simulink model "Microgrid202510141004"  (R2025a)
settings: Solver=ode23tb  StartTime=0  StopTime=2592000  FixedStep=3600  MaxStep=3600  MinStep=1e-4  RelTol=1e-4  AbsTol=1e-6
StartFcn:
  | fprintf('=== Starting Episode [%s] ===\n', datestr(now, 'HH:MM:SS'));
undefined symbols (not defined in the file): D1, Delta
libraries: spsThreePhaseDynamicLoadLib x3, fuzblock x2, spsThreePhaseVIMeasurementLib x2, simulink x1, spsThreePhaseSeriesRLCLoadLib x1, rllib x1, spsThreePhaseTransformerTwoWindingsLib x1, spsThreePhaseBreakerLib x1, spsThreePhaseSourceLib x1, sps_lib x1
settings Model: DataTypeOverride=Off  Creator=jlesage  LastModifiedBy=86138
settings SolverCC: InitialStep=0.1  ZcThreshold=1e-12  AlgebraicLoopSolver=TrustRegion
settings DataIOCC: SaveState=on  ReturnWorkspaceOutputs=off
settings OptimizationCC: OptimizeBlockIOStorage=off  OptimizeDataStoreBuffers=off  BusAssignmentInplaceUpdate=off
settings DebuggingCC: SigSpecEnsureSampleTimeMsg=none  SFUnexpectedBacktrackingDiag=warning  SFNoUnconditionalDefaultTransitionDiag=warning  ArithmeticOperatorsInVariantConditions=warning
settings ModelReferenceCC: EnableRefExpFcnMdlSchedulingChecks=on
settings SFSimCC: SimUseLocalCustomCode=off  CustomCodeUndefinedFunction=UseInterfaceOnly
settings RTWCC: GenCodeOnly=on  GenerateReport=on  RTWUseLocalCustomCode=off  BuildConfiguration=Debug  LaunchReport=on  GPUComputeCapability=3.5
settings CodeAppCC: ForceParamTrailComments=on  MATLABSourceComments=on  EnableCustomComments=on
settings GRTTargetCC: MultiInstanceErrorCode=Warning  CombineSignalStateStructs=on  SupportVariableSizeSignals=on

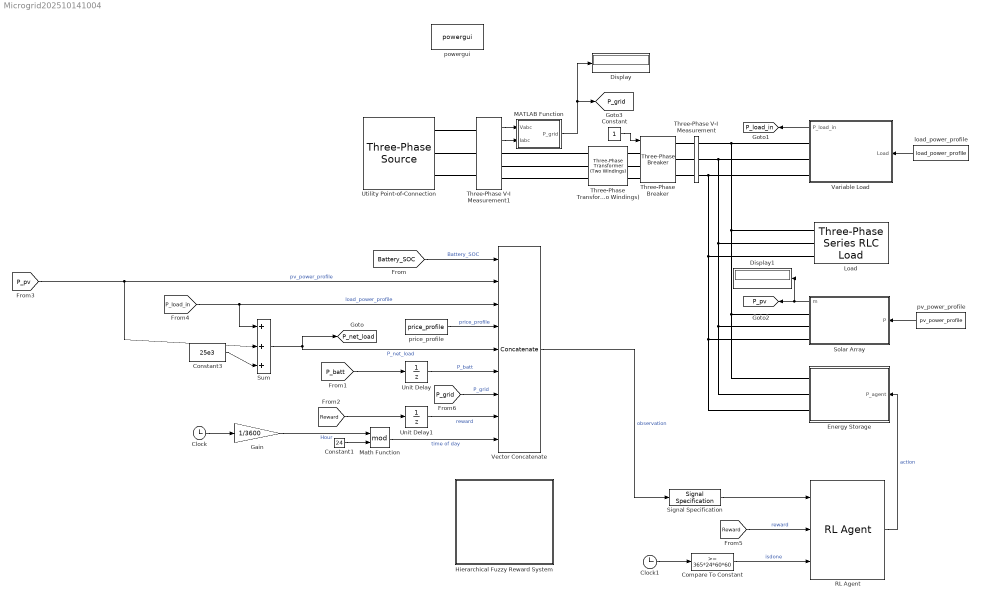
== system Microgrid202510141004 ==
  Clock : Clock
  Clock1 : Clock
  Compare To Constant : simulink/Logic and Bit Operations/Compare To Constant  relop=>=  const=365*24*60*60  OutDataTypeStr=boolean
  Constant : Constant
  Constant1 : Constant  Value=24
  Constant3 : Constant  Value=25e3
  Display : Display
  Display1 : Display
  Energy Storage : Subsystem  mask{Capacity_Ah=280, Fn=60, Vn=400}
      mask prompts: Capacity_Ah "Capacity_Ah of Battery"; Fn "Nominal Frequency [Hz]"; Vn "Nominal L-L Voltage [Vrms]"
      mask DialogControl ParameterGroupVar Prompt: 参数
  Gain : Gain  Gain=1/3600
  Hierarchical Fuzzy Reward System : Subsystem
  Load : spsThreePhaseSeriesRLCLoadLib/Three-Phase Series RLC Load  LConnTagsString=A|B|C  Configuration=Y (grounded)  NominalVoltage=400  Vabc=[1e3 1e3 1e3]  Vabcp=[1e3 1e3 1e3]  NominalFrequency=60  UnbalancedPower=off  ActivePower=25e3  InductivePower=0  CapacitivePower=0  Pabc=[10e3 9e3 11e3]  QLabc=[100 90 110]  QCabc=[100 90 110]  Pabcp=[10e3 9e3 11e3]  QLabcp=[100 90 110]  QCabcp=[100 90 110]  Measurements=None  LoadType=constant Z
      settings: AttributesFormatString=P = %<ActivePower> W
  MATLAB Function : MATLAB Function  TreatAsAtomicUnit=on
  Math Function : Math  Operator=mod
  RL Agent : rllib/RL Agent  Agent=agentObj  ExternalActionAsInput=off  ProvideLastAction=off  ProvideCumRwd=off  TreatAsDirectFeedthrough=on  UseStrictObservationDataTypes=off
  Signal Specification : SignalSpecification  Dimensions=9  SampleTime=3600
  Solar Array : Subsystem  mask(Grid-Connected PV Array (PQ Model)){Vn=400, Fn=60}
      mask prompts: Vn "Nominal L-L Voltage [Vrms]"; Fn "Nominal Frequency [Hz]"
      mask help:
      | This block models a grid-connected solar array using the Three-Phase Dynamic Load block. This is a system-level model that does not contain any power electronics, but is useful for load flow, phasor, and hybrid phasor-EMT simulations. The input to this block is the power output of the grid connected PV array, not irradiance.
      |
      | For more detailed PV models, consider the PV Array block in the Renewables library. Consider using this PQ Model to perform load flow studies and switch to a more detailed model when full EMT studies are required.
      |
      | Note: The array power must be specified for use for Load Flow analysis.
      mask Display:
      | color('white')
      | port_label('input',1,'P')
      | port_label('output',1,'m')
      | port_label('Rconn',1,'A')
      | port_label('Rconn',2,'B')
      | port_label('Rconn',3,'C')
  Sum : Sum  Inputs=+++|
  Three-Phase Transformer (Two Windings) : spsThreePhaseTransformerTwoWindingsLib/Three-Phase Transformer (Two Windings)  Winding1Connection=Delta (D1)  Winding2Connection=Yg  CoreType=Three single-phase transformers  SetSaturation=off  Hysteresis=off  DataFile='hysteresis'  SetInitialFlux=off  Measurements=None  UNITS=pu  NominalPower=[ 100e3, 60 ]  Winding1=[ 13.8e3 , 0.002 , 0.08 ]  Winding2=[ 400 , 0.002 , 0.08 ]  Rm=500  Lm=500  L0=0.5  Saturation=[ 0,0 ; 0.0024,1.2 ; 1.0,1.52 ]  InitialFluxes=[ 0.8 , -0.8 , 0.7 ]  BreakLoop=off  DiscreteSolver=Trapezoidal iterative  DataType=off  TransfoNumber=1
  Three-Phase V-I Measurement : spsThreePhaseVIMeasurementLib/Three-Phase V-I Measurement  VoltageMeasurement=phase-to-ground  SetLabelV=on  LabelV=Vabc  Vpu=off  VpuLL=off  CurrentMeasurement=yes  SetLabelI=on  LabelI=Iabc  Ipu=off  Pbase=100e6  Vbase=500e3  OutputType=Complex  PhasorSimulation=on  PSBequivalent=0
  Three-Phase V-I Measurement1 : spsThreePhaseVIMeasurementLib/Three-Phase V-I Measurement  VoltageMeasurement=phase-to-ground  SetLabelV=off  LabelV=Vabc  Vpu=off  VpuLL=off  CurrentMeasurement=yes  SetLabelI=off  LabelI=Iabc  Ipu=off  Pbase=100e6  Vbase=500e3  OutputType=Complex  PhasorSimulation=on  PSBequivalent=0
  Three-Phase Breaker : spsThreePhaseBreakerLib/Three-Phase Breaker  InitialState=closed  SwitchA=on  SwitchB=on  SwitchC=on  SwitchTimes="[1/60  5/60]"  External=on  BreakerResistance=0.01  SnubberResistance=1e6  SnubberCapacitance=inf  Measurements=None
  Unit Delay : UnitDelay  SampleTime=-1  HasFrameUpgradeWarning=on
  Unit Delay1 : UnitDelay  SampleTime=-1  HasFrameUpgradeWarning=on
  Utility Point-of-Connection : spsThreePhaseSourceLib/Three-Phase Source  InternalConnection=Yg  VoltagePhases=off  Voltage=(13800)*1.00243  PhaseAngle=0.071468  Voltage_phases=[25e3 25e3 25e3]/sqrt(3)  PhaseAngles_phases=[0 -120 +120]  Frequency=60  NonIdealSource=on  SpecifyImpedance=on  Resistance=0.8929  Inductance=16.58e-3  ShortCircuitLevel=250e6  BaseVoltage=13.8e3  XRratio=7  BusType=swing  Pref=10e3  Qref=0  Prefabc=[10e3, 10e3, 10e3]  Qrefabc=[0, 0, 0]  Qmin=-inf  Qmax=inf
  Variable Load : Subsystem  mask(Variable Load (PQ Model)){Vn=400, Fn=60}
      mask prompts: Vn "Nominal L-L Voltage [Vrms]"; Fn "Nominal Frequency [Hz]"
      mask help:
      | The Variable Load block is a lumped approximation for a distribution feeder. For non-unity power factor loads, the input (active power) is scaled accordingly to generate a desired load.
      |
      | Note: The initial input load must be specified for use for Load Flow analysis.
      mask Display:
      | color('white')
      | port_label('input',1,'Load')
      | port_label('Rconn',1,'A')
      | port_label('Rconn',2,'B')
      | port_label('Rconn',3,'C')
  Vector Concatenate : Concatenate  NumInputs=9
  load_power_profile : FromWorkspace  VariableName=load_power_profile  SampleTime=3600
  powergui : sps_lib/powergui  Priority=1  SimulationMode=Phasor  SampleTime=1e-4  frequency=60  Iterations=50  frequencyindice=60  Pbase=100e6  ErrMax=0.0001  UnitsV=kV  UnitsW=MW  buscounter=3  FunctionMessages=off  echomessages=off  EnableUseOfTLC=off  CurrentSourceSwitches=off  DisableSnubberDevices=off  DisableRonSwitches=off  DisableVfSwitches=off  DisplayEquations=off  AutomaticDiscreteSolvers=off  SolverType=Tustin/Backward Euler (TBE)  Interpol=off  ExternalGateDelay=off  methode=off  Ts=100  x0status=blocks  SPID=on  SwTol=0  HookPort=off  NonlinearTolerance=1e-4  nMaxIteration=100  ContinueOnMaxIteration=off  RestoreLinks=warning  ResistiveCurrentMeasurement=off  Frange=[0:2:500]  Ylog=off  Xlog=on  ShowGrid=off  save=off  variable=ZData  structure=0  ZoomFFT=off  StartTime=0.0  cycles=1  DisplayStyle=1  fundamental=60  FreqAxis=off  MaxFrequency=1000  frequencyindicesteady=1  RmsSteady=1  display=off
  price_profile : FromWorkspace  VariableName=price_profile  SampleTime=3600
  pv_power_profile : FromWorkspace  VariableName=pv_power_profile  SampleTime=3600
  tag scope: P_grid=global, P_load_in=global, P_net_load=global, P_pv=global
  wires:
  Constant/1 -> Three-Phase Breaker/1
  pv_power_profile/1 -> Solar Array/1(P)
  load_power_profile/1 -> Variable Load/1(Load)
  Solar Array/1(m) -> [P_pv], Display1/1
  Vector Concatenate/1 -> Signal Specification/1  "observation"
  Clock/1 -> Gain/1
  [Reward] -> RL Agent/2  "reward"
  Compare To Constant/1 -> RL Agent/3  "isdone"
  Clock1/1 -> Compare To Constant/1
  price_profile/1 -> Vector Concatenate/4  "price_profile"
  Gain/1 -> Math Function/1  "Hour"
  [Battery_SOC] -> Vector Concatenate/1  "Battery_SOC"
  [P_pv] -> Sum/2, Vector Concatenate/2  "pv_power_profile"
  [P_load_in] -> Sum/1, Vector Concatenate/3  "load_power_profile"
  Sum/1 -> Vector Concatenate/5, [P_net_load]  "P_net_load"
  [P_batt] -> Unit Delay/1
  [Reward] -> Unit Delay1/1
  Math Function/1 -> Vector Concatenate/9  "time of day"
  Constant1/1 -> Math Function/2
  Unit Delay1/1 -> Vector Concatenate/8  "reward"
  Constant3/1 -> Sum/3
  Variable Load/1(P_load_in) -> [P_load_in]
  Three-Phase V-I Measurement1/1 -> MATLAB Function/1(Vabc)
  Three-Phase V-I Measurement1/2 -> MATLAB Function/2(Iabc)
  MATLAB Function/1(P_grid) -> Display/1, [P_grid]
  Unit Delay/1 -> Vector Concatenate/6  "P_batt"
  [P_grid] -> Vector Concatenate/7  "P_grid"
  Signal Specification/1 -> RL Agent/1
  RL Agent/1 -> Energy Storage/1(P_agent)  "action"
  connections:
  Three-Phase Transformer (Two Windings)/RConn1 -- Three-Phase Breaker/LConn1
  Three-Phase Transformer (Two Windings)/RConn2 -- Three-Phase Breaker/LConn2
  Three-Phase Transformer (Two Windings)/RConn3 -- Three-Phase Breaker/LConn3
  Load/LConn1 -- Three-Phase V-I Measurement/RConn1 -- Variable Load/RConn1 -- Energy Storage/RConn1 -- Solar Array/RConn1
  Load/LConn2 -- Three-Phase V-I Measurement/RConn2 -- Variable Load/RConn2 -- Energy Storage/RConn2 -- Solar Array/RConn2
  Load/LConn3 -- Three-Phase V-I Measurement/RConn3 -- Variable Load/RConn3 -- Energy Storage/RConn3 -- Solar Array/RConn3
  Three-Phase Breaker/RConn1 -- Three-Phase V-I Measurement/LConn1
  Three-Phase Breaker/RConn2 -- Three-Phase V-I Measurement/LConn2
  Three-Phase Breaker/RConn3 -- Three-Phase V-I Measurement/LConn3
  Three-Phase V-I Measurement1/LConn1 -- Utility Point-of-Connection/RConn1
  Three-Phase V-I Measurement1/LConn2 -- Utility Point-of-Connection/RConn2
  Three-Phase V-I Measurement1/LConn3 -- Utility Point-of-Connection/RConn3
  Three-Phase V-I Measurement1/RConn3 -- Three-Phase Transformer (Two Windings)/LConn3
  Three-Phase V-I Measurement1/RConn2 -- Three-Phase Transformer (Two Windings)/LConn2
  Three-Phase V-I Measurement1/RConn1 -- Three-Phase Transformer (Two Windings)/LConn1

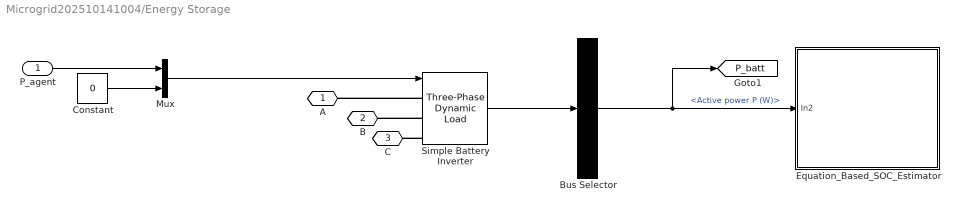
== system Microgrid202510141004/Energy Storage ==
  P_agent : Inport
  Bus Selector : BusSelector  OutputSignals=Active power P (W)
  Constant : Constant  Value=0
  Equation_Based_SOC_Estimator : Subsystem
  Mux : Mux  Inputs=2
  Simple Battery Inverter : spsThreePhaseDynamicLoadLib/Three-Phase Dynamic Load  NominalVoltage=[Vn Fn]  ActiveReactivePowers=[-100000 -3.38813e-13]  PositiveSequence=[0.999844 -0.0038635]  ExternalControl=on  NpNq=[1.3 2]  TimeConstants="[0  0  0  0]"  MinimumVoltage=0.7  Tfilter=1e-2  LoadFlowParameters=[4,0,0,0,0]
      settings: LibrarySourceBlock=|
      | sps_lib/Passives/Three-Phase
      | Dynamic Load
  A : PMIOPort  Side=Right
  B : PMIOPort  Port=2  Side=Right
  C : PMIOPort  Port=3  Side=Right
  tag scope: P_batt=global
  wires:
  Simple Battery Inverter/1 -> Bus Selector/1
  Bus Selector/1 -> [P_batt], Equation_Based_SOC_Estimator/1(In2)  "<Active power P (W)>"
  Mux/1 -> Simple Battery Inverter/1
  P_agent/1 -> Mux/1
  Constant/1 -> Mux/2
  connections:
  Simple Battery Inverter/LConn1 -- A/RConn1
  Simple Battery Inverter/LConn2 -- B/RConn1
  Simple Battery Inverter/LConn3 -- C/RConn1

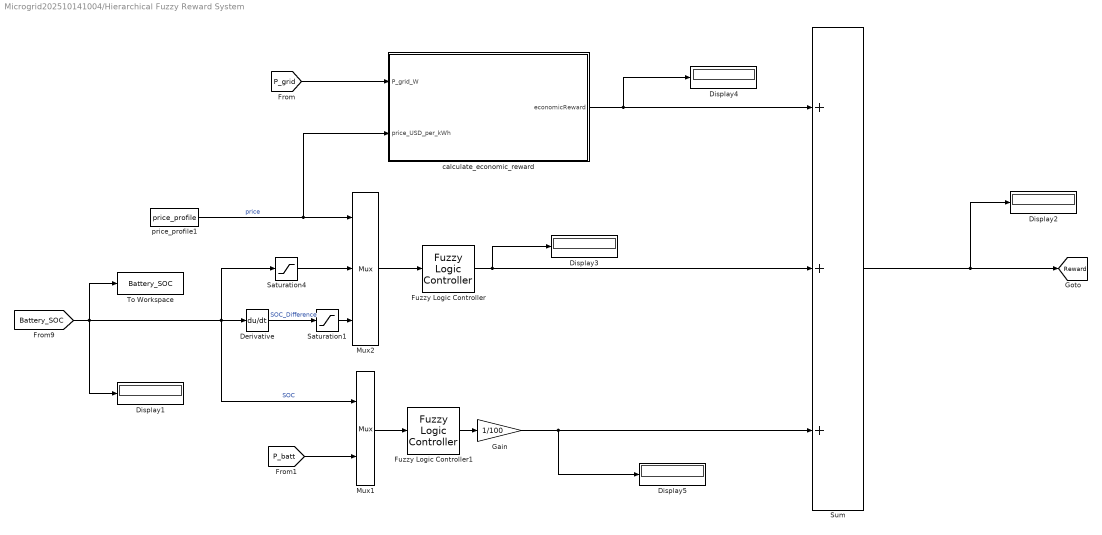
== system Microgrid202510141004/Hierarchical Fuzzy Reward System ==
  Derivative : Derivative
  Display{1..5} (5 alike) : Display
  Fuzzy Logic Controller : fuzblock/Fuzzy Logic  Controller  FIS='Battery_State_Type2.fis'  OutputSampleNumber=101  DataType=double  UseLookupTable=off  NumBreakpoints=10  FuzzifiedInputs=off  RuleFiringStrengths=off  RuleOutputs=off  AggregatedOutputs=off  SimulateUsing=Interpreted execution  OutOfRangeInputValueMessage=warning  NoRuleFiredMessage=warning  EmptyOutputFuzzySetMessage=warning
  Fuzzy Logic Controller1 : fuzblock/Fuzzy Logic  Controller  FIS='SOCProtector_Type2.fis'  OutputSampleNumber=101  DataType=double  UseLookupTable=off  NumBreakpoints=10  FuzzifiedInputs=off  RuleFiringStrengths=off  RuleOutputs=off  AggregatedOutputs=off  SimulateUsing=Interpreted execution  OutOfRangeInputValueMessage=warning  NoRuleFiredMessage=warning  EmptyOutputFuzzySetMessage=warning
  Gain : Gain  Gain=1/100
  Mux1 : Mux  Inputs=2
  Mux2 : Mux  Inputs=3
  Saturation1 : Saturate  UpperLimit=100  LowerLimit=-100  LinearizeAsGain=off  ZeroCross=off  OutMin=-100  RndMeth=Simplest
  Saturation4 : Saturate  UpperLimit=100  LowerLimit=0  LinearizeAsGain=off  ZeroCross=off  OutMin=0  RndMeth=Simplest
  Sum : Sum  Inputs=+++
  To Workspace : ToWorkspace  VariableName=Battery_SOC  SampleTime=3600
      settings: Save2DSignal=2-D array (concatenate along first dimension)
  calculate_economic_reward : MATLAB Function  TreatAsAtomicUnit=on
  price_profile1 : FromWorkspace  VariableName=price_profile
  tag scope: Reward=global
  wires:
  Sum/1 -> Display2/1, [Reward]
  Mux2/1 -> Fuzzy Logic Controller/1
  [Battery_SOC] -> Display1/1, To Workspace/1, Derivative/1, Mux1/1, Saturation4/1  "SOC"
  Derivative/1 -> Saturation1/1  "SOC_Difference"
  Saturation4/1 -> Mux2/2
  [P_grid] -> calculate_economic_reward/1(P_grid_W)
  price_profile1/1 -> calculate_economic_reward/2(price_USD_per_kWh), Mux2/1  "price"
  calculate_economic_reward/1(economicReward) -> Sum/1, Display4/1
  Fuzzy Logic Controller/1 -> Display3/1, Sum/2
  Mux1/1 -> Fuzzy Logic Controller1/1
  Fuzzy Logic Controller1/1 -> Gain/1
  [P_batt] -> Mux1/2
  Gain/1 -> Display5/1, Sum/3
  Saturation1/1 -> Mux2/3

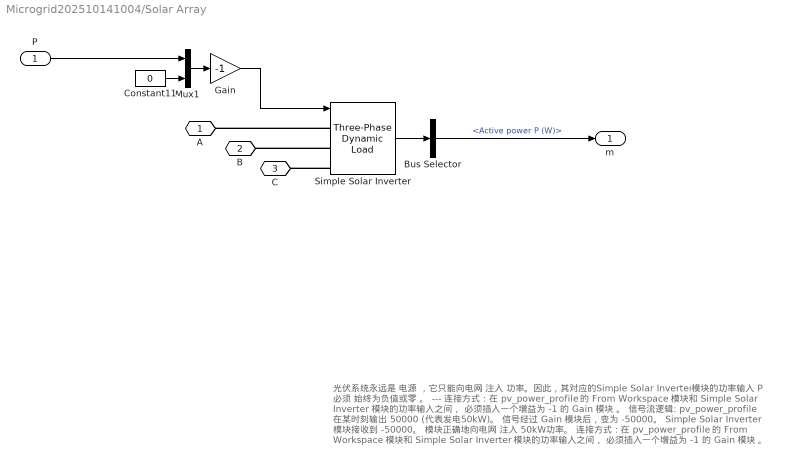
== system Microgrid202510141004/Solar Array ==
  note: 光伏系统永远是 电源 ，它只能向电网 注入 功率。因此，其对应的Simple Solar Inverter模块的功率输入 P 必须 始终为负值或零 。
      |
      | ---
      |
      | 连接方式 : 在 pv_power_profile 的 From Workspace 模块和 Simple Solar Inverter 模块的功率输入之间， 必须插入一个增益为 -1 的 Gain 模块 。
      | 信号流逻辑: pv_power_profile 在某时刻输出 50000 (代表发电50kW)。
      | 信号经过 Gain 模块后，变为 -50000。
      | Simple Solar Inverter 模块接收到 -50000。
      | 模块正确地向电网 注入 50kW功率。 连接方式 : 在 pv_power_profile 的 From Workspace 模块和 Simple Solar Inverter 模块的功率输入之间， 必须插入一个增益为 -1 的 Gain 模块 。
  P : Inport
  Bus Selector : BusSelector  OutputSignals=Active power P (W)
  Constant11 : Constant  Value=0
  Gain : Gain  Gain=-1
  Mux1 : Mux  Inputs=2
  Simple Solar Inverter : spsThreePhaseDynamicLoadLib/Three-Phase Dynamic Load  NominalVoltage=[Vn Fn]  ActiveReactivePowers=[-12000 0]  PositiveSequence=[0.999844 -0.0038635]  ExternalControl=on  NpNq=[1.3 2]  TimeConstants="[0  0  0  0]"  MinimumVoltage=0.7  Tfilter=1e-2  LoadFlowParameters=[4,0,0,0,0]
      settings: LibrarySourceBlock=|
      | sps_lib/Passives/Three-Phase
      | Dynamic Load
  A : PMIOPort  Side=Right
  B : PMIOPort  Port=2  Side=Right
  C : PMIOPort  Port=3  Side=Right
  m : Outport  VectorParamsAs1DForOutWhenUnconnected=off
  wires:
  P/1 -> Mux1/1
  Mux1/1 -> Gain/1
  Constant11/1 -> Mux1/2
  Simple Solar Inverter/1 -> Bus Selector/1
  Bus Selector/1 -> m/1  "<Active power P (W)>"
  Gain/1 -> Simple Solar Inverter/1
  connections:
  Simple Solar Inverter/LConn2 -- B/RConn1
  Simple Solar Inverter/LConn3 -- C/RConn1
  Simple Solar Inverter/LConn1 -- A/RConn1

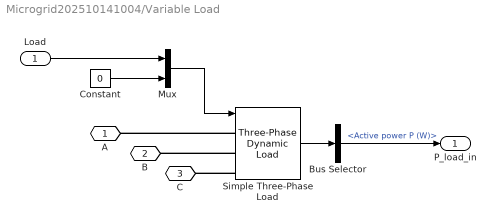
== system Microgrid202510141004/Variable Load ==
  Load : Inport
  Bus Selector : BusSelector  OutputSignals=Active power P (W)
  Constant : Constant  Value=0
  Mux : Mux  Inputs=2
  Simple Three-Phase Load : spsThreePhaseDynamicLoadLib/Three-Phase Dynamic Load  NominalVoltage=[Vn Fn]  ActiveReactivePowers=[200000 0.1]  PositiveSequence=[0.999844 -0.0038635]  ExternalControl=on  NpNq=[1.3 2]  TimeConstants="[0  0  0  0]"  MinimumVoltage=0.7  Tfilter=1e-2  LoadFlowParameters=[4,0,0,0,0]
      settings: LibrarySourceBlock=|
      | sps_lib/Passives/Three-Phase
      | Dynamic Load
  A : PMIOPort  Side=Right
  B : PMIOPort  Port=2  Side=Right
  C : PMIOPort  Port=3  Side=Right
  P_load_in : Outport
  wires:
  Simple Three-Phase Load/1 -> Bus Selector/1
  Mux/1 -> Simple Three-Phase Load/1
  Load/1 -> Mux/1
  Constant/1 -> Mux/2
  Bus Selector/1 -> P_load_in/1  "<Active power P (W)>"
  connections:
  Simple Three-Phase Load/LConn1 -- A/RConn1
  Simple Three-Phase Load/LConn3 -- C/RConn1
  Simple Three-Phase Load/LConn2 -- B/RConn1

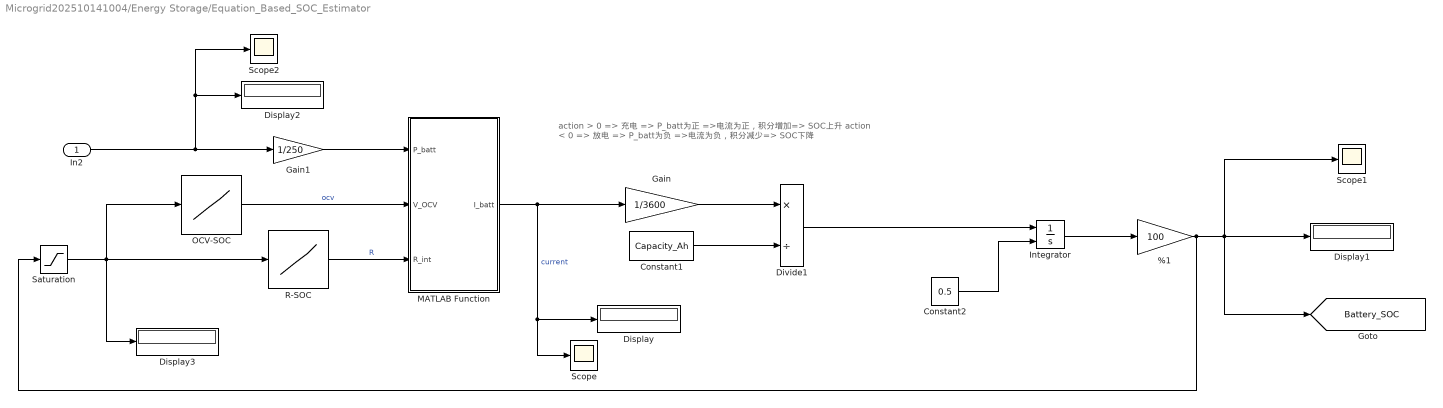
== system Microgrid202510141004/Energy Storage/Equation_Based_SOC_Estimator ==
  note: action > 0 => 充电 => P_batt为正 =>电流为正，积分增加=> SOC上升
      | action < 0 => 放电 => P_batt为负 =>电流为负，积分减少=> SOC下降
  In2 : Inport
  %1 : Gain  Gain=100
  Constant1 : Constant  Value=Capacity_Ah
  Constant2 : Constant  Value=0.5
  Display{,1..3} (4 alike) : Display
  Divide1 : Product  Inputs=*/
  Gain : Gain  Gain=1/3600
  Gain1 : Gain  Gain=1/250
  Integrator : Integrator  InitialConditionSource=external
  MATLAB Function : MATLAB Function  TreatAsAtomicUnit=on
  OCV-SOC : Lookup_n-D  NumberOfTableDimensions=1  BreakpointsForDimension1=[0;1;5;10;20;30;40;50;60;70;80;90;95;99;100]  Table=[2.5;2.73;2.9;3;3.2;3.22;3.25;3.26;3.27;3.3;3.32;3.35;3.4;3.5;3.65]  InternalRulePriority=Speed  RndMeth=Simplest
  R-SOC : Lookup_n-D  NumberOfTableDimensions=1  BreakpointsForDimension1=[0;1;5;10;20;30;40;50;60;70;80;90;95;99;100]  Table=[0.0005999999999999999;0.0005;0.00045;0.0004;0.00035;0.00025;0.0002;0.00018;0.00018;0.00019;0.0002;0.00022;0.00025;0.00035;0.0004]  InternalRulePriority=Speed  RndMeth=Simplest
  Saturation : Saturate  UpperLimit=100  LowerLimit=0
  Scope : Scope
      settings: ActiveDisplayYMinimum=-8.6273114509056246  ActiveDisplayYMaximum=-8.6266897894405368
  Scope1 : Scope
      settings: ActiveDisplayYMinimum=-151.94347281099479  ActiveDisplayYMaximum=296.21727807075712
  Scope2 : Scope
      settings: ActiveDisplayYMinimum=-14040.738664657363  ActiveDisplayYMaximum=-6783.8632493780851  DataLoggingVariableName=ScopeData2
  tag scope: Battery_SOC=global
  wires:
  Gain/1 -> Divide1/1
  %1/1 -> Saturation/1, [Battery_SOC], Scope1/1, Display1/1
  Divide1/1 -> Integrator/1
  Integrator/1 -> %1/1
  Constant2/1 -> Integrator/2
  OCV-SOC/1 -> MATLAB Function/2(V_OCV)  "ocv"
  Constant1/1 -> Divide1/2
  R-SOC/1 -> MATLAB Function/3(R_int)  "R"
  Gain1/1 -> MATLAB Function/1(P_batt)
  Saturation/1 -> Display3/1, R-SOC/1, OCV-SOC/1
  MATLAB Function/1(I_batt) -> Gain/1, Scope/1, Display/1  "current"
  In2/1 -> Gain1/1, Scope2/1, Display2/1

== matlab function Microgrid202510141004/Energy Storage/Equation_Based_SOC_Estimator/MATLAB Function ==
  data: P_batt input; V_OCV input; R_int input; I_batt output
function I_batt = fcn(P_batt, V_OCV, R_int)
% =========================================================================
% 功能: 根据单电芯功率、开路电压和内阻计算电池电流
% 模型: V_term = V_OCV + I_batt * R_int (一阶ECM)
% -------------------------------------------------------------------------
% 输入:
%   P_batt: 单个电芯的功率 (W)。
%           (注意: 这是从系统总功率缩放后的值)
%   V_OCV:  当前SOC下的单电芯开路电压 (V)。
%   R_int:  当前SOC和SOH下的单电芯等效内阻 (Ohm)。
% -------------------------------------------------------------------------
% 输出:
%   I_batt: 计算出的单电芯电流 (A)。
% =========================================================================

    % 物理方程推导:
    % 1) P_batt = V_term * I_batt
    % 2) V_term = V_OCV + I_batt * R_int  =>  I_batt = (V_term - V_OCV) / R_int
    % 将 (2) 代入 (1):
    % P_batt = V_term * (V_term - V_OCV) / R_int
    % 整理得到关于 V_term 的一元二次方程:
    % V_term^2 - V_OCV * V_term - P_batt * R_int = 0

    % -- 步骤 1: 计算一元二次方程的判别式 --
    % 判别式 delta = b^2 - 4ac, 其中 a=1, b=-V_OCV, c=-P_batt*R_int
    discriminant = V_OCV^2 + 4 * P_batt * R_int;

    % -- 步骤 2: 检查解的物理可行性 --
    % 如果判别式小于0，意味着在当前 V_OCV 和 R_int 条件下，电池无法
    % 提供或吸收这么大的功率，方程没有实数解。这通常发生在请求的
    % 放电功率超过了电池的最大输出功率 P_max = V_OCV^2 / (4*R_int)。
    % 在这种情况下，我们将电流视为0，模拟BMS的功率限制行为。
    if discriminant < 0
        I_batt = 0; % 功率请求超出物理极限，返回0电流
        % 在实际应用中，此处可以增加一个警告标志输出
        return; % 提前退出函数
    end

    % -- 步骤 3: 求解端电压 V_term --
    % 根据求根公式 V_term = (-b ± sqrt(delta)) / 2a
    % V_term = (V_OCV ± sqrt(discriminant)) / 2
    % 我们需要选择物理上有意义的解。
    % 充电时 (P_batt > 0), V_term > V_OCV。
    % 放电时 (P_batt < 0), V_term < V_OCV。
    % 经过分析，使用 "+" 号的解在两种情况下都能满足物理约束。
    V_term = (V_OCV + sqrt(discriminant)) / 2;

    % -- 步骤 4: 计算电流 I_batt --
    % 为避免当 R_int 极小时可能出现的数值不稳定问题，我们进行一个简单的检查。
    if R_int < 1e-6 % 避免除以一个非常小的数或零
        % 如果内阻几乎为0, 则 V_term 约等于 V_OCV。
        if abs(V_OCV) > 1e-6
            I_batt = P_batt / V_OCV;
        else
            I_batt = 0; % V_OCV也为0，无法计算
        end
    else
        % 使用 V_term = V_OCV + I_batt * R_int 的变形公式计算电流。
        % 这比 I_batt = P_batt / V_term 在数值上更稳定。
        I_batt = (V_term - V_OCV) / R_int;
    end
end

== matlab function Microgrid202510141004/MATLAB Function ==
  data: Vabc input; P_grid output; Iabc input
function P_grid = fcn(Vabc, Iabc)
% =========================================================================
% 功能: 根据三相复数电压和电流计算总有功功率
% 模型: S = V * conj(I), P = real(S_total)
% -------------------------------------------------------------------------
% 输入:
%   Vabc: 3x1的复数电压向量 [Va; Vb; Vc] (Phasor in RMS)
%   Iabc: 3x1的复数电流向量 [Ia; Ib; Ic] (Phasor in RMS)
% -------------------------------------------------------------------------
% 输出:
%   P_grid: 三相总有功功率 (W)
% =========================================================================

    % 确保输入是列向量，以保证计算的稳健性
    Vabc = Vabc(:);
    Iabc = Iabc(:);

    % 1. 计算每相的复功率 (Element-wise multiplication)
    %    S_per_phase = [Va*conj(Ia); Vb*conj(Ib); Vc*conj(Ic)]
    S_per_phase = Vabc .* conj(Iabc);

    % 2. 将三相复功率相加得到总复功率
    S_total = sum(S_per_phase);

    % 3. 提取总复功率的实部，即为总有功功率
    P_grid = real(S_total);

end

== matlab function Microgrid202510141004/Hierarchical Fuzzy Reward System/calculate_economic_reward ==
  data: P_grid_W input; economicReward output; price_USD_per_kWh input
function economicReward = calculate_economic_reward(P_grid_W, price_USD_per_kWh)
%CALCULATE_ECONOMIC_REWARD Compute the economic reward component.
%   economicReward = CALCULATE_ECONOMIC_REWARD(P_grid_W, price_USD_per_kWh)
%   returns the reward associated with buying or selling power at the
%   current price. Positive values represent revenue, negative values
%   represent cost. Internal constants determine penalty strength.
%
%   Inputs:
%       P_grid_W          - Grid exchange power [W], >0 buy, <0 sell.
%       price_USD_per_kWh - Real-time energy price [$/kWh].
%
%   Output:
%       economicReward    - Scalar economic reward contribution.

    arguments
        P_grid_W (1,1) double
        price_USD_per_kWh (1,1) double
    end

    % Tunable constants (adjust in code if needed).
    peakPowerThresholdW = 15e3;  % [W] Peak import threshold.
    highPriceThreshold = 0.40;   % [$/kWh] High price definition.
    penaltyFactor = 5e-8;        % Quadratic penalty scale.
    timeStepHours = 1.0;         % Simulation step duration [h].

    % Core transaction term: revenue when exporting, cost when importing.
    P_grid_kW = P_grid_W / 1000.0;
    linear_reward = -(P_grid_kW * price_USD_per_kWh * timeStepHours);

    % Peak power penalty discourages expensive peak-hour imports.
    peak_penalty = 0.0;
    if (P_grid_W > 0) && (P_grid_W > peakPowerThresholdW) && (price_USD_per_kWh > highPriceThreshold)
        peak_penalty = -penaltyFactor * (P_grid_W ^ 2);
    end

    economicReward = linear_reward + peak_penalty;
end
